simulink model "d_2PSKyangyanruiMATLAB7"  (Simulink 6.0)
settings: Solver=ode45  StartTime=0.0  StopTime=10  RelTol=1e-3
libraries: commchan2 x1, dsparch4 x1, commrandsrc2 x1, commsink2 x1, dspsnks4 x1, dspsigops x1
settings Model: LastModifiedBy=xxgcxy602  BufferReuse=off
settings OptimizationCC: BlockReduction=off  InlineParams=on  BufferReuse=off

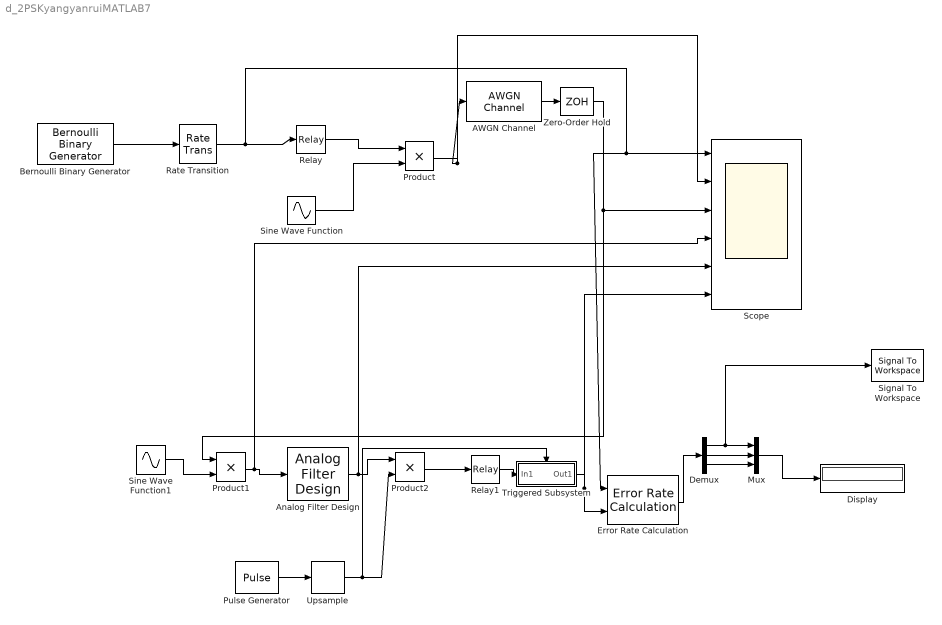
== system d_2PSKyangyanruiMATLAB7 ==
  AWGN Channel : commchan2/AWGN Channel  seed=67  noiseMode="Signal to noise ratio  (SNR)"  EbNodB=10  EsNodB=10  SNRdB=10  bitsPerSym=1  Ps=1  Tsym=1  variance=1
  Analog Filter Design : dsparch4/Analog Filter Design  method=Butterworth  filttype=Lowpass  N=2  Wlo=2*pi  Whi=80  Rp=2  Rs=40
  Bernoulli Binary Generator : commrandsrc2/Bernoulli Binary Generator  P=0.5  seed=61  Ts=1  frameBased=off  sampPerFrame=1  orient=off
  Demux : Demux  Outputs=3
  Display : Display
  Error Rate Calculation : commsink2/Error Rate Calculation  N=0  st_delay=0  cp_mode=Entire frame  subframe=[]  PMode=Port  WsName=ErrorVec  RsMode2=off  stop=off  numErr=100  maxBits=1e6
  Mux : Mux  Inputs=3
  Product : Product  RndMeth=Zero
  Product1 : Product  RndMeth=Zero
  Product2 : Product  RndMeth=Zero
  Pulse Generator : DiscretePulseGenerator  Period=10  PulseWidth=3  SampleTime=1/50
  Rate Transition : RateTransition
  Relay : Relay  OnSwitchValue=0.1  OffSwitchValue=0.1  OffOutputValue=-1
  Relay1 : Relay  OnSwitchValue=0.1  OffSwitchValue=0.1
  Scope : Scope  NumInputPorts=6
      settings: YMin=-5~-5~-5~-5~-5~-5  YMax=5~5~5~5~5~5
  Signal To Workspace : dspsnks4/Signal To Workspace  VariableName=ERRout  FrameMode=Concatenate frames (2-D array)
      settings: FixptAsFi=off
  Sine Wave Function : Sin  Bias=2*pi*2  SampleTime=1/500
  Sine Wave Function1 : Sin  Bias=2*pi*2  SampleTime=1/500
  Triggered Subsystem : Subsystem  TreatAsAtomicUnit=on
  Upsample : dspsigops/Upsample  N=1  phase=0  ic=0  mode=Maintain input frame size
  Zero-Order Hold : ZeroOrderHold  SampleTime=1/500
  wires:
  Bernoulli Binary Generator/1 -> Rate Transition/1
  Rate Transition/1 -> Relay/1, Error Rate Calculation/1, Scope/1
  Relay/1 -> Product/1
  Sine Wave Function/1 -> Product/2
  Product/1 -> AWGN Channel/1, Scope/2
  Sine Wave Function1/1 -> Product1/2
  Product1/1 -> Analog Filter Design/1, Scope/4
  Pulse Generator/1 -> Upsample/1
  Analog Filter Design/1 -> Product2/1, Scope/5
  Product2/1 -> Relay1/1
  Upsample/1 -> Product2/2, Triggered Subsystem/Trigger
  Demux/1 -> Mux/1, Signal To Workspace/1
  Demux/2 -> Mux/2
  Demux/3 -> Mux/3
  Mux/1 -> Display/1
  Relay1/1 -> Triggered Subsystem/1(In1)
  Triggered Subsystem/1(Out1) -> Error Rate Calculation/2, Scope/6
  AWGN Channel/1 -> Zero-Order Hold/1
  Zero-Order Hold/1 -> Product1/1, Scope/3
  Error Rate Calculation/1 -> Demux/1

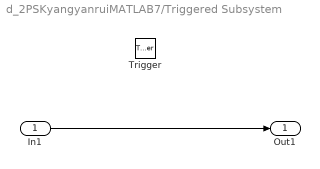
== system d_2PSKyangyanruiMATLAB7/Triggered Subsystem ==
  In1 : Inport  Port=1  LatchInput=off
  Trigger : TriggerPort
  Out1 : Outport
  wires:
  In1/1 -> Out1/1
